simulink model "sat_orbit_orientation"  (R2019b)
settings: Solver=ode45  StartTime=0.0  StopTime=15000.0  MaxStep=0.009  RelTol=1e-8
libraries: simulink x1
settings Model: Creator=Hector  LastModifiedBy=Hector
settings SolverCC: AlgebraicLoopSolver=LineSearch

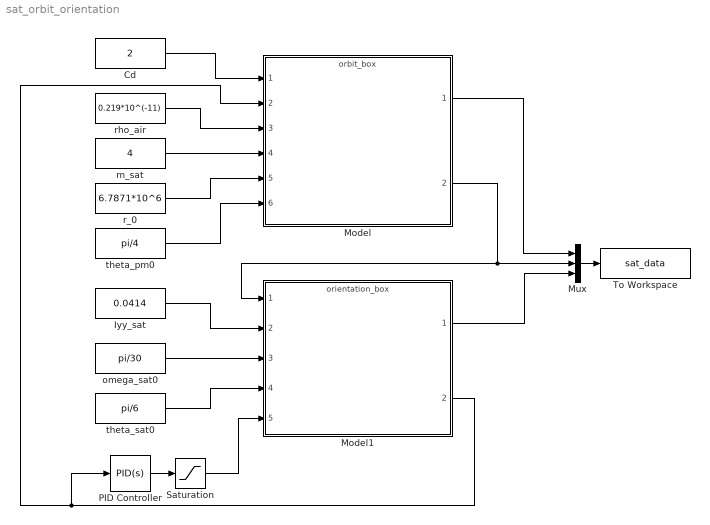
== system sat_orbit_orientation ==
  Cd : Constant  Value=2
  Iyy_sat : Constant  Value=0.0414
  Model : ModelReference  ModelNameDialog=orbit_box.slx  SimulationMode=Normal  ModelReferenceVersion=1.31
  Model1 : ModelReference  ModelNameDialog=orientation_box.slx  SimulationMode=Normal  ModelReferenceVersion=1.29
  Mux : Mux  Inputs=3
  PID Controller : simulink/Continuous/PID Controller  Controller=PID  Form=Parallel  TimeDomain=Continuous-time  SampleTime=-1  IntegratorMethod=Forward Euler  FilterMethod=Forward Euler  ControllerParametersSource=internal  P=5.33827881904527e-05  I=2.08258616091013e-07  D=0.00336002738651377  UseFilter=on  N=0.454497521184683  TunerSelectOption=Transfer Function Based (PID Tuner App)  InitialConditionSource=internal  InitialConditionForIntegrator=0  InitialConditionForFilter=0  DifferentiatorICPrevScaledInput=0  ExternalReset=none  TrackingMode=off  Kt=1  LimitOutput=off  UpperSaturationLimit=inf  LowerSaturationLimit=-inf  LinearizeAsGain=on  AntiWindupMode=none  Kb=1  POutMin=[]  POutMax=[]  IOutMin=[]  IOutMax=[]  DOutMin=[]  DOutMax=[]  NOutMin=[]  NOutMax=[]  SumOutMin=[]  SumOutMax=[]  SaturationOutMin=[]  SaturationOutMax=[]  PParamMin=[]  PParamMax=[]  IParamMin=[]  IParamMax=[]  DParamMin=[]  DParamMax=[]  NParamMin=[]  NParamMax=[]  KbParamMin=[]  KbParamMax=[]  KtParamMin=[]  KtParamMax=[]  KbOutMin=[]  KbOutMax=[]  KtOutMin=[]  KtOutMax=[]  IntegratorOutMin=[]  IntegratorOutMax=[]  FilterOutMin=[]  FilterOutMax=[]  SumI1OutMin=[]  SumI1OutMax=[]  SumI2OutMin=[]  SumI2OutMax=[]  SumI3OutMin=[]  SumI3OutMax=[]  SumI4OutMin=[]  SumI4OutMax=[]  SumDOutMin=[]  SumDOutMax=[]  DifferentiatorOutMin=[]  DifferentiatorOutMax=[]  FilterDiffOutCoefMin=[]  FilterDiffOutCoefMax=[]  ReciprocalOutMin=[]  ReciprocalOutMax=[]  SumDenOutMin=[]  SumDenOutMax=[]  SumNumOutMin=[]  SumNumOutMax=[]  DivideOutMin=[]  DivideOutMax=[]  IntegratorContinuousStateAttributes=''  IntegratorStateMustResolveToSignalObject=off  IntegratorRTWStateStorageClass=Auto  FilterContinuousStateAttributes=''  FilterStateMustResolveToSignalObject=off  FilterRTWStateStorageClass=Auto  ParallelPVariant=InternalParameters  IdealPVariant=Disabled  IVariant=InternalParameters  DVariant=InternalParameters  IntegratorVariant=Continuous  SatVariant=Disabled  AWVariant=Passthrough  PCopyVariant=Disabled  TRVariant=Disabled  FdbkBlocksVariant=Forward  IdealPFdbkVariant=Disabled  SatFdbkVariant=Disabled  DerivativeFilterVariant=ContFilter  NVariant=InternalParameters  NCopyVariant=Disabled  FilterICVariant=InternalICsFilter  IntegratorICVariant=InternalICs  ExternalResetVariant=Disabled  TRSumVariant=Passthrough  SumFdbkVariant=Disabled  SumVariant=Sum_PID
  Saturation : Saturate  UpperLimit=0.00023  LowerLimit=-0.00023
  To Workspace : ToWorkspace  VariableName=sat_data  SampleTime=-1
  m_sat : Constant  Value=4
  omega_sat0 : Constant  Value=pi/30
  r_0 : Constant  Value=6.7871*10^6
  rho_air : Constant  Value=0.219*10^(-11)
  theta_pm0 : Constant  Value=pi/4
  theta_sat0 : Constant  Value=pi/6
  wires:
  Cd/1 -> Model/1
  Model1/2 -> Model/2, PID Controller/1
  rho_air/1 -> Model/3
  m_sat/1 -> Model/4
  r_0/1 -> Model/5
  theta_pm0/1 -> Model/6
  Model/2 -> Mux/2, Model1/1
  Iyy_sat/1 -> Model1/2
  omega_sat0/1 -> Model1/3
  theta_sat0/1 -> Model1/4
  PID Controller/1 -> Saturation/1
  Saturation/1 -> Model1/5
  Model/1 -> Mux/1
  Mux/1 -> To Workspace/1
  Model1/1 -> Mux/3
